simulink model "simu_theo1_converter"  (R2018a)
settings: Solver=ode1  StartTime=0.0  StopTime=10.0  FixedStep=1e-6  RelTol=1e-3
values from neighbouring files (symbols this model uses):
  A = dsys.A    [affine_TimeVar_Ex1.m]    (also in h2_project.m = [-R/L  -1/L; h2_project_pid.m = [-R/L  -1/L; limit_cycle - Copia.m; limit_cycle.m)
  x0 = xe_h{1}    [affine_TimeVar_Ex1.m]    (also in general_circuit.m = [0; 0]; limit_cycle - Copia.m; limit_cycle.m; main.m = [0; 0])
settings Model: Creator=julio  LastModifiedBy=julio

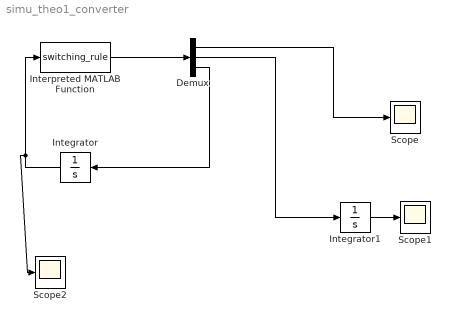
== system simu_theo1_converter ==
  Demux : Demux  Outputs=[1 1 length(A{1})]
  Integrator : Integrator  InitialCondition=x0
  Integrator1 : Integrator
  Interpreted MATLAB Function : MATLABFcn  MATLABFcn=switching_rule
  Scope : Scope
  Scope1 : Scope
  Scope2 : Scope
  wires:
  Interpreted MATLAB Function/1 -> Demux/1
  Integrator/1 -> Scope2/1, Interpreted MATLAB Function/1
  Demux/3 -> Integrator/1
  Demux/2 -> Integrator1/1
  Demux/1 -> Scope/1
  Integrator1/1 -> Scope1/1
